simulink model "LAB2_Pendulum"  (R2022b)
settings: Solver=FixedStepAuto  StartTime=t0  StopTime=tf  FixedStep=0.1  RelTol=1e-3
values from neighbouring files (symbols this model uses):
  g = 9.81    [LAB_02.m]
  l = 5    [LAB_02.m]
  theta0 = 0    [LAB_02.m]
  theta_dot0 = pi/4    (= 0.785398163397)    [LAB_02.m]
settings Model: Creator=ludov  LastModifiedBy=ludov

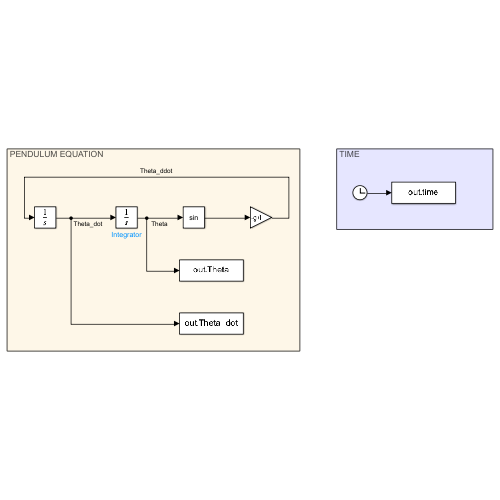
[thumbnail: Simulink's stored preview of the top-level diagram]
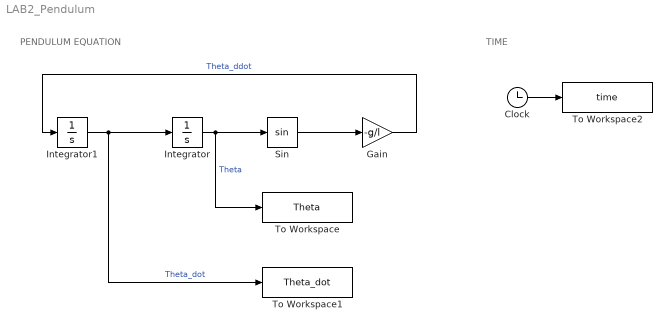
== system LAB2_Pendulum ==
  note: PENDULUM EQUATION
  note: TIME
  Clock : Clock
  Gain : Gain  Gain=-g/l
  Integrator : Integrator  InitialCondition=theta0
  Integrator1 : Integrator  InitialCondition=theta_dot0
  Sin : Trigonometry
  To Workspace : ToWorkspace  VariableName=Theta  SaveFormat=Timeseries  SampleTime=-1
  To Workspace1 : ToWorkspace  VariableName=Theta_dot  SaveFormat=Timeseries  SampleTime=-1
  To Workspace2 : ToWorkspace  VariableName=time  SaveFormat=Timeseries  SampleTime=-1
  wires:
  Integrator/1 -> Sin/1, To Workspace/1  "Theta"
  Integrator1/1 -> To Workspace1/1, Integrator/1  "Theta_dot"
  Sin/1 -> Gain/1
  Gain/1 -> Integrator1/1  "Theta_ddot"
  Clock/1 -> To Workspace2/1
